simulink model "StateSpaceM"  (R2014b)
settings: Solver=ode45  StartTime=0.0  StopTime=10.0  RelTol=1e-3
settings Model: Creator=99641  LastModifiedBy=99641

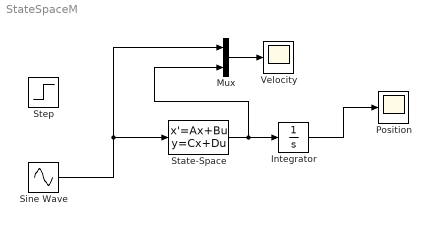
== system StateSpaceM ==
  Integrator : Integrator
  Mux : Mux  Inputs=2
  "Position " : Scope
  Sine Wave : Sin  SampleTime=0
  State-Space : StateSpace  A=[0,1;-5,0]  B=[0;10]  C=[1,0]  D=0  X0=0
  Step : Step  SampleTime=0
  Velocity : Scope
  wires:
  Integrator/1 -> "Position "/1
  State-Space/1 -> Mux/2, Integrator/1
  Sine Wave/1 -> Mux/1, State-Space/1
  Mux/1 -> Velocity/1
